simulink model "mainmodel"  (R2014a)
settings: Solver=ode45  StartTime=0.0  StopTime=10.0  RelTol=1e-3
libraries: powerlib x6, powerlib_meascontrol x1
settings Model: Creator=hsinwang  LastModifiedBy=hsinwang

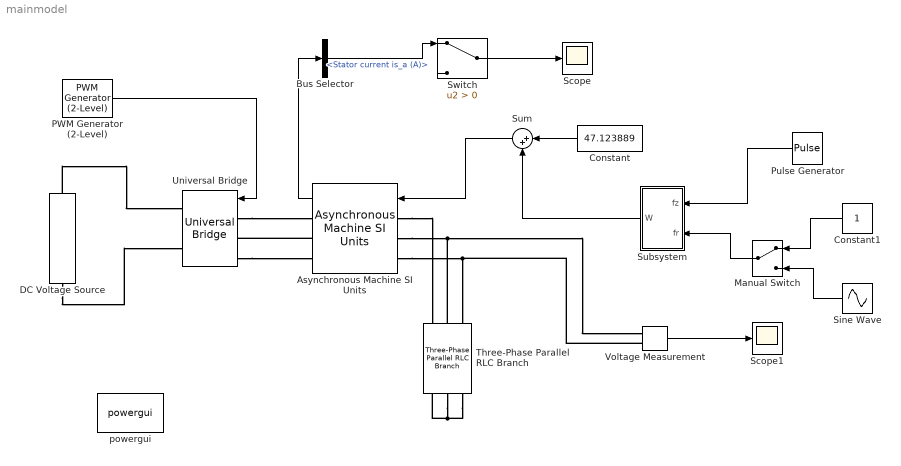
== system mainmodel ==
  Asynchronous Machine SI Units : powerlib/Machines/Asynchronous Machine SI Units  PresetModel=No  MechanicalLoad=Speed w  ShowDetailedParameters=on  RotorType=Wound  ReferenceFrame=Rotor  Units=SI  MeasurementBus=off  NominalParameters=[3000 380 60]  Stator=[1.9188 0.2412]  Rotor=[2.5712 0.2412]  Cage1=[ 0.022 0.226/377]  Cage2=[ 0.022 0.226/377]  Lm=0.2340  Mechanical=[0.4 0.02187 2]  PolePairs=2  InitialConditions=[1 0 0 0 0 0 0 0]  SimulateSaturation=off  Saturation=[14.03593122, 27.81365428, 53.79336849, 72.68890987, 97.98006896, 148.6815601, 215.7428561, 302.9841135, 420.4778367 ; 230, 322, 414, 460, 506, 552, 598, 644, 690]  LoadFlowParameters=1492000  TsPowergui=0  TsBlock=-1  IterativeModel=Trapezoidal non iterative  Pmec=0
  Bus Selector : BusSelector  OutputSignals=Stator measurements.Stator current is_a (A)
  Constant : Constant  Value=47.123889
  Constant1 : Constant
  DC Voltage Source : powerlib/Electrical Sources/DC Voltage Source  Amplitude=100  Measurements=None
  Manual Switch : ManualSwitch
  PWM Generator (2-Level) : powerlib_meascontrol/Pulse & Signal Generators/PWM Generator (2-Level)  ModulatorType=Three-phase bridge (6 pulses)  ModulatorMode=Unsynchronized  nF=27  Fc=27*60  ModulatingSignals=off  m=0.8  Freq=60  Phase=0  Ts=0
  Pulse Generator : DiscretePulseGenerator  PulseType=Time based  Period=10  PulseWidth=5  SampleTime=2
  Scope : Scope
      settings: YMin=-3.5e-15  YMax=3.5e-15
  Scope1 : Scope
      settings: TickLabels=on  YMin=-5.5e-15  YMax=5.5e-15
  Sine Wave : Sin  SampleTime=0
  Subsystem : Subsystem
  Sum : Sum  Inputs=|++
  Switch : Switch  Criteria=u2 > Threshold
  Three-Phase Parallel RLC Branch : powerlib/Elements/Three-Phase Parallel RLC Branch  LConnTagsString=A|B|C  RConnTagsString=A|B|C  BranchType=R  Resistance=1  Inductance=1e-3  Capacitance=1e-6  Measurements=None
  Universal Bridge : powerlib/Power Electronics/Universal Bridge  Arms=3  SnubberResistance=1e5  SnubberCapacitance=inf  Device=IGBT / Diodes  Ron=1e-3  Lon=0  ForwardVoltages="[  0  0  ]"  ForwardVoltage=0  GTOparameters=[ 10e-6 , 20e-6 ]  IGBTparameters=[ 1e-6 , 2e-6 ]  Measurements=None  Measurements_2=None  converterType=Rectifier
  Voltage Measurement : powerlib/Measurements/Voltage Measurement  PhasorSimulation=off  OutputType=Complex  PSBequivalent=0
  powergui : powerlib/powergui  Priority=1  SimulationMode=Continuous  SolverType=Tustin  SampleTime=50e-6  frequency=60  SPID=off  DisableSnubberDevices=off  DisableRonSwitches=off  DisableVfSwitches=off  SwTol=0  Interpol=off  DisplayEquations=off  Ts=0  methode=off  frequencyindice=60  Pbase=1e6  ErrMax=1e-4  Iterations=50  UnitsV=V  UnitsW=kW  FunctionMessages=off  echomessages=off  HookPort=off  EnableUseOfTLC=off  x0status=blocks  RestoreLinks=warning  ResistiveCurrentMeasurement=off  Frange=[0:2:500]  Ylog=off  Xlog=on  ShowGrid=off  save=off  variable=ZData  structure=0  ZoomFFT=off  StartTime=0.0  cycles=1  DisplayStyle=1  fundamental=60  FreqAxis=off  MaxFrequency=1000  frequencyindicesteady=1  RmsSteady=1  display=off
  wires:
  PWM Generator (2-Level)/1 -> Universal Bridge/1
  Bus Selector/1 -> Switch/1  "<Stator current is_a (A)>"
  Voltage Measurement/1 -> Scope1/1
  Constant/1 -> Sum/1
  Constant1/1 -> Manual Switch/1
  Sine Wave/1 -> Manual Switch/2
  Subsystem/1(W) -> Sum/2
  Manual Switch/1 -> Subsystem/2("fr ")
  Pulse Generator/1 -> Subsystem/1("fz ")
  Asynchronous Machine SI Units/1 -> Bus Selector/1
  Sum/1 -> Asynchronous Machine SI Units/1
  Switch/1 -> Scope/1
  connections:
  DC Voltage Source/RConn1 -- Universal Bridge/RConn1
  DC Voltage Source/LConn1 -- Universal Bridge/RConn2
  Three-Phase Parallel RLC Branch/LConn3 -- Three-Phase Parallel RLC Branch/LConn2 -- Three-Phase Parallel RLC Branch/LConn1
  Three-Phase Parallel RLC Branch/RConn2 -- Voltage Measurement/LConn1 -- Asynchronous Machine SI Units/LConn2
  Voltage Measurement/LConn2 -- Asynchronous Machine SI Units/LConn3 -- Three-Phase Parallel RLC Branch/RConn3
  Universal Bridge/LConn1 -- Asynchronous Machine SI Units/RConn1
  Asynchronous Machine SI Units/RConn2 -- Universal Bridge/LConn2
  Universal Bridge/LConn3 -- Asynchronous Machine SI Units/RConn3
  Asynchronous Machine SI Units/LConn1 -- Three-Phase Parallel RLC Branch/RConn1

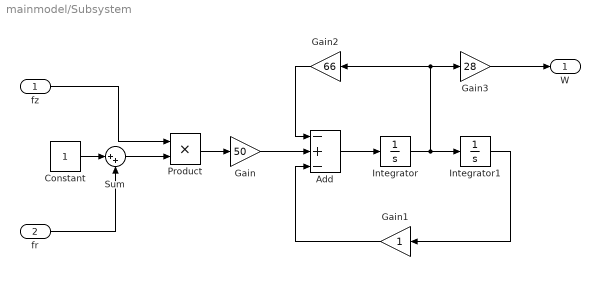
== system mainmodel/Subsystem ==
  "fz " : Inport
  "fr " : Inport  Port=2
  Add : Sum  Inputs=-+-
  Constant : Constant
  Gain : Gain  Gain=50
  Gain1 : Gain
  Gain2 : Gain  Gain=66
  Gain3 : Gain  Gain=28
  Integrator : Integrator
  Integrator1 : Integrator
  Product : Product
  Sum : Sum  Inputs=|++
  W : Outport
  wires:
  Gain3/1 -> W/1
  Gain2/1 -> Add/1
  Gain1/1 -> Add/3
  Integrator1/1 -> Gain1/1
  Integrator/1 -> Gain2/1, Gain3/1, Integrator1/1
  Add/1 -> Integrator/1
  Gain/1 -> Add/2
  Product/1 -> Gain/1
  "fz "/1 -> Product/1
  Sum/1 -> Product/2
  "fr "/1 -> Sum/2
  Constant/1 -> Sum/1
